simulink model "anticipation"  (R2015b)
settings: Solver=VariableStepAuto  StartTime=0.0  StopTime=30  RelTol=1e-3
values from neighbouring files (symbols this model uses):
  K = (Kd^2)/4    (= 2.25)    [commande_robot.m]
  Kd = 3    [commande_robot.m]
  r = R(1)    [commande_robot.m]    (also in sf_loi_avant_RP.m; sf_retour_linearisant_RP.m)
libraries: lib_robotRP x3
settings Model: Creator=chamand  LastModifiedBy=chamand

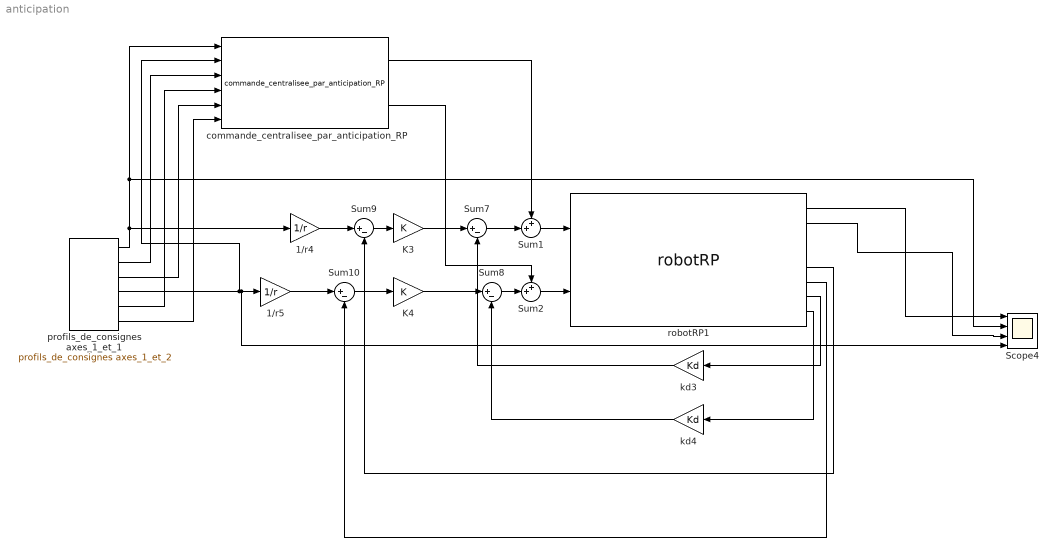
== system anticipation ==
  1/r4 : Gain  Gain=1/r
  1/r5 : Gain  Gain=1/r
  K3 : Gain  Gain=K
  K4 : Gain  Gain=K
  Scope4 : Scope  NumInputPorts=4
  Sum1 : Sum  Inputs=++|
  Sum{7..10} (4 alike) : Sum  Inputs=|+-
  Sum2 : Sum  Inputs=++|
  commande_centralisee_par_anticipation_RP : lib_robotRP/commande_centralisee_par_anticipation_RP  SystemSampleTime=-1
  kd3 : Gain  Gain=Kd
  kd4 : Gain  Gain=Kd
  profils_de_consignes axes_1_et_1 : lib_robotRP/profils_de_consignes axes_1_et_2
  robotRP1 : lib_robotRP/robotRP  vecteur_theta_dtheta_initial=[0 ; 1/2/r ; 0 ; 0]  m=15  gX=0  gY=-9.81  F1=0  F2=0  H1=0  H2=0  Km_sur_R=0.3  Jm=0.01  Beff=0.0125  r=1/200
  wires:
  kd3/1 -> Sum7/2
  robotRP1/7 -> kd3/1
  robotRP1/5 -> Sum9/2
  robotRP1/1 -> Scope4/1
  Sum9/1 -> K3/1
  robotRP1/2 -> Scope4/3
  robotRP1/8 -> kd4/1
  robotRP1/6 -> Sum10/2
  Sum10/1 -> K4/1
  kd4/1 -> Sum8/2
  K3/1 -> Sum7/1
  K4/1 -> Sum8/1
  profils_de_consignes axes_1_et_1/1 -> 1/r4/1, Scope4/2, commande_centralisee_par_anticipation_RP/1
  profils_de_consignes axes_1_et_1/4 -> commande_centralisee_par_anticipation_RP/2, Scope4/4, 1/r5/1
  1/r5/1 -> Sum10/1
  1/r4/1 -> Sum9/1
  Sum1/1 -> robotRP1/1
  Sum2/1 -> robotRP1/2
  Sum8/1 -> Sum2/2
  Sum7/1 -> Sum1/2
  commande_centralisee_par_anticipation_RP/1 -> Sum1/1
  commande_centralisee_par_anticipation_RP/2 -> Sum2/1
  profils_de_consignes axes_1_et_1/2 -> commande_centralisee_par_anticipation_RP/3
  profils_de_consignes axes_1_et_1/5 -> commande_centralisee_par_anticipation_RP/4
  profils_de_consignes axes_1_et_1/3 -> commande_centralisee_par_anticipation_RP/5
  profils_de_consignes axes_1_et_1/6 -> commande_centralisee_par_anticipation_RP/6
